simulink model "MiniProject"  (R2020a)
settings: Solver=VariableStepAuto  StartTime=0.0  StopTime=10.0  RelTol=1e-3
values from neighbouring files (symbols this model uses):
  angVelPerVolt = 12/255    (= 0.0470588235294)    [MiniProjectScript.m]
  K = 12/255    (= 0.0470588235294)    [MiniProject2_Controller.m]    (also in MiniProjectScript.m)
  sig = 22    [MiniProject2_Controller.m]    (also in MiniProjectScript.m)
settings Model: Creator=brett  LastModifiedBy=brett

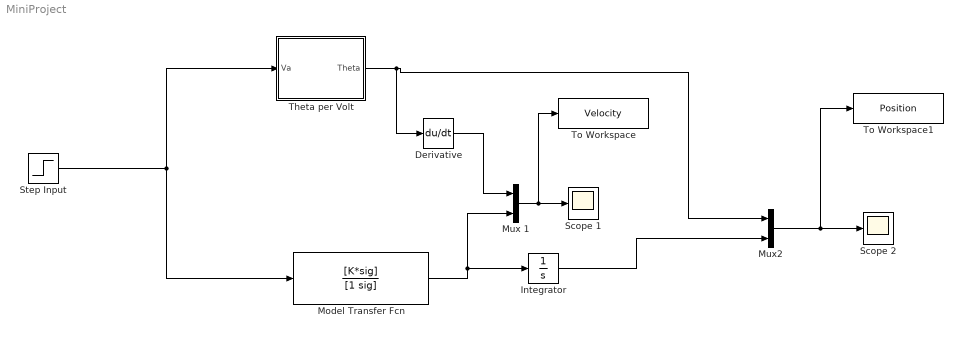
== system MiniProject ==
  Derivative : Derivative
  Integrator : Integrator
  Model Transfer Fcn : TransferFcn  Numerator=[K*sig]  Denominator=[1 sig]
  Mux 1 : Mux  Inputs=2
  Mux2 : Mux  Inputs=2
  Scope 1 : Scope
  Scope 2 : Scope
  Step Input : Step  After=255  SampleTime=0
  Theta per Volt : Subsystem
  To Workspace : ToWorkspace  VariableName=Velocity  SaveFormat=Timeseries  SampleTime=-1
  To Workspace1 : ToWorkspace  VariableName=Position  SaveFormat=Timeseries  SampleTime=-1
  wires:
  Mux2/1 -> To Workspace1/1, Scope 2/1
  Step Input/1 -> Model Transfer Fcn/1, Theta per Volt/1(Va)
  Mux 1/1 -> To Workspace/1, Scope 1/1
  Integrator/1 -> Mux2/2
  Model Transfer Fcn/1 -> Mux 1/2, Integrator/1
  Theta per Volt/1(Theta) -> Derivative/1, Mux2/1
  Derivative/1 -> Mux 1/1

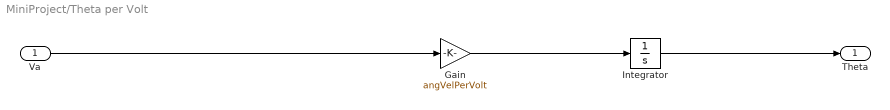
== system MiniProject/Theta per Volt ==
  Va : Inport
  Gain : Gain  Gain=angVelPerVolt
  Integrator : Integrator
  Theta : Outport
  wires:
  Va/1 -> Gain/1
  Gain/1 -> Integrator/1
  Integrator/1 -> Theta/1
